simulink model "dao_dong_tu_kich"  (R2023a)
settings: Solver=ode4  StartTime=0.0  StopTime=50  FixedStep=0.001  RelTol=1e-3
settings Model: Creator=VINH  LastModifiedBy=VINH

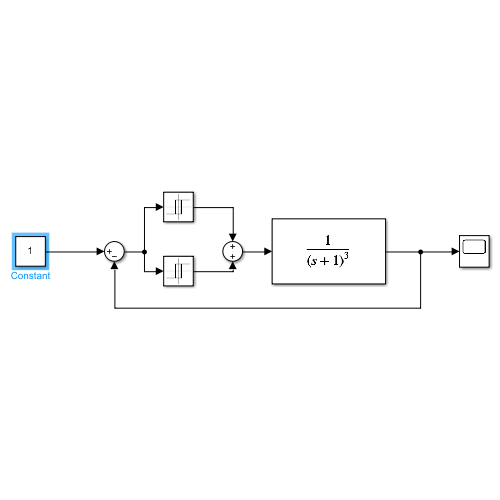
[thumbnail: Simulink's stored preview of the top-level diagram]
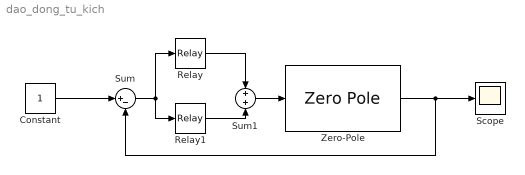
== system dao_dong_tu_kich ==
  Constant : Constant
  Relay : Relay  OnSwitchValue=0.5  OffSwitchValue=0.5  OnOutputValue=10
  Relay1 : Relay  OnSwitchValue=-0.5  OffSwitchValue=-0.5  OnOutputValue=0  OffOutputValue=-10
  Scope : Scope
  Sum : Sum  Inputs=|+-
  Sum1 : Sum  Inputs=+|+
  Zero-Pole : ZeroPole  Zeros=[]  Poles=[-1 -1 -1]  Gain=1
  wires:
  Constant/1 -> Sum/1
  Sum/1 -> Relay1/1, Relay/1
  Zero-Pole/1 -> Sum/2, Scope/1
  Relay/1 -> Sum1/1
  Relay1/1 -> Sum1/2
  Sum1/1 -> Zero-Pole/1
